simulink model "untitled"  (R2018b)
settings: Solver=VariableStepAuto  StartTime=0.0  StopTime=inf  RelTol=1e-3
undefined symbols (not defined in the file or in its folder): Angular, Linear
libraries: robotlib x3, sharedtransform x1
settings Model: EnablePacing=on  Creator=raffaele  LastModifiedBy=raffaele

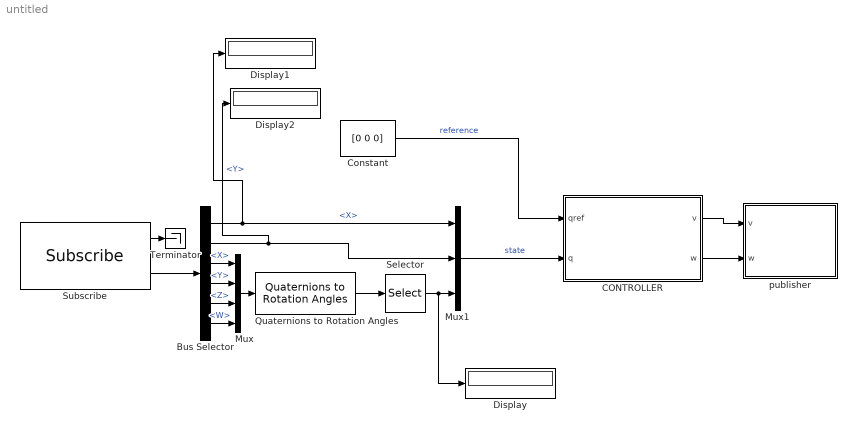
== system untitled ==
  Bus Selector : BusSelector  OutputSignals=Pose.Pose.Position.X,Pose.Pose.Position.Y,Pose.Pose.Orientation.X,Pose.Pose.Orientation.Y,Pose.Pose.Orientation.Z,Pose.Pose.Orientation.W
  CONTROLLER : MATLAB Function  TreatAsAtomicUnit=on
  Constant : Constant  Value=[0 0 0]
  Display : Display
  Display1 : Display
  Display2 : Display
  Mux : Mux
  Mux1 : Mux  Inputs=3
  Quaternions to Rotation Angles : sharedtransform/Quaternions to Rotation Angles  rotationOrder=ZYX  aMode=aMode
      settings: SourceProductBaseCode=AE
  Selector : Selector  InputPortWidth=3  IndexOptions=Index vector (dialog)  Indices=3  OutputSizes=1
  Subscribe : robotlib/Subscribe  topicSource=Select from ROS network  topic=/odometry/filtered  messageType=nav_msgs/Odometry  sampleTime=-1  messageQueueLength=1
      settings: SourceProductBaseCode=RO
  Terminator : Terminator
  publisher : Subsystem
  wires:
  Subscribe/1 -> Terminator/1
  Subscribe/2 -> Bus Selector/1
  Bus Selector/3 -> Mux/1  "<X>"
  Bus Selector/4 -> Mux/2  "<Y>"
  Bus Selector/5 -> Mux/3  "<Z>"
  Bus Selector/6 -> Mux/4  "<W>"
  Mux/1 -> Quaternions to Rotation Angles/1
  Bus Selector/2 -> Display2/1, Mux1/2  "<Y>"
  Bus Selector/1 -> Display1/1, Mux1/1  "<X>"
  Quaternions to Rotation Angles/1 -> Selector/1
  Mux1/1 -> CONTROLLER/2(q)  "state"
  Selector/1 -> Display/1, Mux1/3
  Constant/1 -> CONTROLLER/1(qref)  "reference"
  CONTROLLER/1(v) -> publisher/1(v)
  CONTROLLER/2(w) -> publisher/2(w)

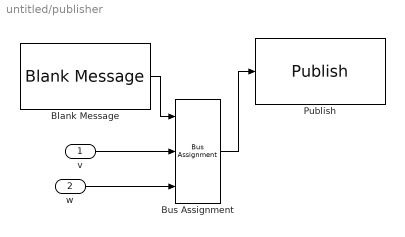
== system untitled/publisher ==
  v : Inport
  w : Inport  Port=2
  Blank Message : robotlib/Blank Message  messageClass=Message  entityType=geometry_msgs/Twist  messageType=geometry_msgs/Twist  SampleTime=inf
      settings: SourceProductBaseCode=RO
  Bus Assignment : BusAssignment  AssignedSignals=Linear.X,Angular.Z
  Publish : robotlib/Publish  topicSource=Select from ROS network  topic=/husky_velocity_controller/cmd_vel  messageType=geometry_msgs/Twist  messageQueueLength=1
      settings: SourceProductBaseCode=RO
  wires:
  Blank Message/1 -> Bus Assignment/1
  v/1 -> Bus Assignment/2
  w/1 -> Bus Assignment/3
  Bus Assignment/1 -> Publish/1

== matlab function untitled/CONTROLLER ==
  data: qref input; q input; v output; w output
function [v,w] = controller(qref,q)
x=q(1); xref=qref(1);
y=q(2); yref=qref(2);
th=q(3); thref = qref(3);

v = xref-x;
w = thref-th;

% k1=1;
% k2=0.1;
% k3=0;
% v =  k1*((xref-x)*cos(th) +(yref-y)* sin(th));
% w = k2*(atan2((yref-y),(xref-x)) - th + pi );

% ro = sqrt((xref-x).^2 + (yref-y).^2);
% gamma = atan2((yref-y),(xref-x)) - th +pi;
% delta = gamma + th;
% v = k1*ro*cos(gamma);
% w = k2*gamma + k1*(sin(gamma)*cos(gamma)/gamma)*(gamma+k3*delta);
